simulink model "test_mdl"  (R2018a)
settings: Solver=VariableStepAuto  StartTime=0.0  StopTime=10.0  RelTol=1e-3
(part 7 of 8)

== system test_mdl/FD1_CAN_P702_GASD_MY21_DCV_V06/PCM_HEV/Cluster_HEV_Data5 ==
  HybMdeStat_D_Dsply : Constant
  PlgActvArb_B_Dsply : Constant
  bus_creator : BusCreator  Inputs=2
  port : Outport
  wires:
  bus_creator/1 -> port/1  "Cluster_HEV_Data5"
  HybMdeStat_D_Dsply/1 -> bus_creator/1  "HybMdeStat_D_Dsply"
  PlgActvArb_B_Dsply/1 -> bus_creator/2  "PlgActvArb_B_Dsply"

== system test_mdl/FD1_CAN_P702_GASD_MY21_DCV_V06/PCM_HEV/DCACA_Data4 ==
  DcacElPw_D_Stat : Constant
  DcacEngOnMsgTxt_D_Rq : Constant
  DcacFaltMsgTxt_D_Rq : Constant
  DcacGfciTest_B_Rq : Constant
  DcacHw_D_Confg : Constant
  DcacLedCtl_D_Rq : Constant
  DcacLoFuelMsgTxt_D_Rq : Constant
  DcacOn_B_Rq : Constant
  DcacOut1_Pw_Dsply : Constant
  DcacOut2_Pw_Dsply : Constant
  DcacOut_Pw_DsplyMx : Constant
  DcacSys_B_Falt : Constant
  PwBedPnlEnbl_B_Rq : Constant
  bus_creator : BusCreator  Inputs=13
  port : Outport
  wires:
  bus_creator/1 -> port/1  "DCACA_Data4"
  DcacElPw_D_Stat/1 -> bus_creator/1  "DcacElPw_D_Stat"
  DcacEngOnMsgTxt_D_Rq/1 -> bus_creator/2  "DcacEngOnMsgTxt_D_Rq"
  DcacFaltMsgTxt_D_Rq/1 -> bus_creator/3  "DcacFaltMsgTxt_D_Rq"
  DcacGfciTest_B_Rq/1 -> bus_creator/4  "DcacGfciTest_B_Rq"
  DcacHw_D_Confg/1 -> bus_creator/5  "DcacHw_D_Confg"
  DcacLedCtl_D_Rq/1 -> bus_creator/6  "DcacLedCtl_D_Rq"
  DcacLoFuelMsgTxt_D_Rq/1 -> bus_creator/7  "DcacLoFuelMsgTxt_D_Rq"
  DcacOn_B_Rq/1 -> bus_creator/8  "DcacOn_B_Rq"
  DcacOut1_Pw_Dsply/1 -> bus_creator/9  "DcacOut1_Pw_Dsply"
  DcacOut2_Pw_Dsply/1 -> bus_creator/10  "DcacOut2_Pw_Dsply"
  DcacOut_Pw_DsplyMx/1 -> bus_creator/11  "DcacOut_Pw_DsplyMx"
  DcacSys_B_Falt/1 -> bus_creator/12  "DcacSys_B_Falt"
  PwBedPnlEnbl_B_Rq/1 -> bus_creator/13  "PwBedPnlEnbl_B_Rq"

== system test_mdl/FD1_CAN_P702_GASD_MY21_DCV_V06/PCM_HEV/EngBrakeData ==
  AccEngStat_D_Actl : Constant
  AccStopMde_D_Rq : Constant
  BPedDrvAppl_D_QF : Constant
  BpedDrvAppl_D_Actl : Constant
  CcMde_D_Actl : Constant
  CcOvrrdActv_B_Actl : Constant
  CcStat_D_Actl : Constant
  CmbbDeny_B_ActlPrpl : Constant
  CmbbEngTqMn_B_Actl : Constant
  EngAout_N_MnAllw : Constant
  PrplTqMnSat_B_Actl : Constant
  Veh_V_DsplyCcSet : Constant
  bus_creator : BusCreator  Inputs=12
  port : Outport
  wires:
  bus_creator/1 -> port/1  "EngBrakeData"
  AccEngStat_D_Actl/1 -> bus_creator/1  "AccEngStat_D_Actl"
  AccStopMde_D_Rq/1 -> bus_creator/2  "AccStopMde_D_Rq"
  BPedDrvAppl_D_QF/1 -> bus_creator/3  "BPedDrvAppl_D_QF"
  BpedDrvAppl_D_Actl/1 -> bus_creator/4  "BpedDrvAppl_D_Actl"
  CcMde_D_Actl/1 -> bus_creator/5  "CcMde_D_Actl"
  CcOvrrdActv_B_Actl/1 -> bus_creator/6  "CcOvrrdActv_B_Actl"
  CcStat_D_Actl/1 -> bus_creator/7  "CcStat_D_Actl"
  CmbbDeny_B_ActlPrpl/1 -> bus_creator/8  "CmbbDeny_B_ActlPrpl"
  CmbbEngTqMn_B_Actl/1 -> bus_creator/9  "CmbbEngTqMn_B_Actl"
  EngAout_N_MnAllw/1 -> bus_creator/10  "EngAout_N_MnAllw"
  PrplTqMnSat_B_Actl/1 -> bus_creator/11  "PrplTqMnSat_B_Actl"
  Veh_V_DsplyCcSet/1 -> bus_creator/12  "Veh_V_DsplyCcSet"

== system test_mdl/FD1_CAN_P702_GASD_MY21_DCV_V06/PCM_HEV/EngVehicleSpThrottle ==
  ApedPosPcActl_D_Qf : Constant
  ApedPosPcActl_No_Cnt : Constant
  ApedPosPcActl_No_Cs : Constant
  ApedPos_PcRate_ActlArb : Constant
  ApedPos_Pc_ActlArb : Constant
  EngAout3_N_Actl : Constant
  EngAoutNActl_D_QF : Constant
  EngAout_N_Actl : Constant
  bus_creator : BusCreator  Inputs=8
  port : Outport
  wires:
  bus_creator/1 -> port/1  "EngVehicleSpThrottle"
  ApedPosPcActl_D_Qf/1 -> bus_creator/1  "ApedPosPcActl_D_Qf"
  ApedPosPcActl_No_Cnt/1 -> bus_creator/2  "ApedPosPcActl_No_Cnt"
  ApedPosPcActl_No_Cs/1 -> bus_creator/3  "ApedPosPcActl_No_Cs"
  ApedPos_PcRate_ActlArb/1 -> bus_creator/4  "ApedPos_PcRate_ActlArb"
  ApedPos_Pc_ActlArb/1 -> bus_creator/5  "ApedPos_Pc_ActlArb"
  EngAout3_N_Actl/1 -> bus_creator/6  "EngAout3_N_Actl"
  EngAoutNActl_D_QF/1 -> bus_creator/7  "EngAoutNActl_D_QF"
  EngAout_N_Actl/1 -> bus_creator/8  "EngAout_N_Actl"

== system test_mdl/FD1_CAN_P702_GASD_MY21_DCV_V06/PCM_HEV/EngVehicleSpThrottle2 ==
  GearRvrse_D_Actl : Constant
  StrtrMtrCtlMsgTxt_D2_Rq : Constant
  StrtrMtrCtlMsgTxt_D_Rq : Constant
  StrtrMtrDlyStrt_B_Stat : Constant
  VehVActlEng_D_Qf : Constant
  VehVActlEng_No_Cnt : Constant
  VehVActlEng_No_Cs : Constant
  VehVTrlrAid_B_Avail : Constant
  Veh_V_ActlEng : Constant
  Veh_V_RqCcSet : Constant
  bus_creator : BusCreator  Inputs=10
  port : Outport
  wires:
  bus_creator/1 -> port/1  "EngVehicleSpThrottle2"
  GearRvrse_D_Actl/1 -> bus_creator/1  "GearRvrse_D_Actl"
  StrtrMtrCtlMsgTxt_D2_Rq/1 -> bus_creator/2  "StrtrMtrCtlMsgTxt_D2_Rq"
  StrtrMtrCtlMsgTxt_D_Rq/1 -> bus_creator/3  "StrtrMtrCtlMsgTxt_D_Rq"
  StrtrMtrDlyStrt_B_Stat/1 -> bus_creator/4  "StrtrMtrDlyStrt_B_Stat"
  VehVActlEng_D_Qf/1 -> bus_creator/5  "VehVActlEng_D_Qf"
  VehVActlEng_No_Cnt/1 -> bus_creator/6  "VehVActlEng_No_Cnt"
  VehVActlEng_No_Cs/1 -> bus_creator/7  "VehVActlEng_No_Cs"
  VehVTrlrAid_B_Avail/1 -> bus_creator/8  "VehVTrlrAid_B_Avail"
  Veh_V_ActlEng/1 -> bus_creator/9  "Veh_V_ActlEng"
  Veh_V_RqCcSet/1 -> bus_creator/10  "Veh_V_RqCcSet"

== system test_mdl/FD1_CAN_P702_GASD_MY21_DCV_V06/PCM_HEV/EngineClimateData ==
  AirAmbTe_D_Qf : Constant
  AirAmb_P_Actl : Constant
  AirAmb_Te_Actl : Constant
  AirAmb_Te_ActlFilt : Constant
  AslChime_B_Rq : Constant
  AslIconDsply_D_Rq : Constant
  DynoMde_B_Cmd : Constant
  EcssLamp_D_RqDsply : Constant
  EngAout_Aa_Actl : Constant
  GasPrtc_D_RqDsply : Constant
  HvacHtrCore2_Te_Actl : Constant
  bus_creator : BusCreator  Inputs=11
  port : Outport
  wires:
  bus_creator/1 -> port/1  "EngineClimateData"
  AirAmbTe_D_Qf/1 -> bus_creator/1  "AirAmbTe_D_Qf"
  AirAmb_P_Actl/1 -> bus_creator/2  "AirAmb_P_Actl"
  AirAmb_Te_Actl/1 -> bus_creator/3  "AirAmb_Te_Actl"
  AirAmb_Te_ActlFilt/1 -> bus_creator/4  "AirAmb_Te_ActlFilt"
  AslChime_B_Rq/1 -> bus_creator/5  "AslChime_B_Rq"
  AslIconDsply_D_Rq/1 -> bus_creator/6  "AslIconDsply_D_Rq"
  DynoMde_B_Cmd/1 -> bus_creator/7  "DynoMde_B_Cmd"
  EcssLamp_D_RqDsply/1 -> bus_creator/8  "EcssLamp_D_RqDsply"
  EngAout_Aa_Actl/1 -> bus_creator/9  "EngAout_Aa_Actl"
  GasPrtc_D_RqDsply/1 -> bus_creator/10  "GasPrtc_D_RqDsply"
  HvacHtrCore2_Te_Actl/1 -> bus_creator/11  "HvacHtrCore2_Te_Actl"

== system test_mdl/FD1_CAN_P702_GASD_MY21_DCV_V06/PCM_HEV/EngineData_1 ==
  SeatWorkSrfc_B_Falt : Constant
  TrnIpcDsplyGear_D_Actl : Constant
  TrnIpcDsplyGear_D_Stat : Constant
  TrnIpcDsplyMde_D_Actl : Constant
  TrnIpcDsplyMde_D_Stat : Constant
  TrnIpcDsplyRng2_D_Actl : Constant
  TrnIpcDsplyRng_D_Stat : Constant
  bus_creator : BusCreator  Inputs=7
  port : Outport
  wires:
  bus_creator/1 -> port/1  "EngineData_1"
  SeatWorkSrfc_B_Falt/1 -> bus_creator/1  "SeatWorkSrfc_B_Falt"
  TrnIpcDsplyGear_D_Actl/1 -> bus_creator/2  "TrnIpcDsplyGear_D_Actl"
  TrnIpcDsplyGear_D_Stat/1 -> bus_creator/3  "TrnIpcDsplyGear_D_Stat"
  TrnIpcDsplyMde_D_Actl/1 -> bus_creator/4  "TrnIpcDsplyMde_D_Actl"
  TrnIpcDsplyMde_D_Stat/1 -> bus_creator/5  "TrnIpcDsplyMde_D_Stat"
  TrnIpcDsplyRng2_D_Actl/1 -> bus_creator/6  "TrnIpcDsplyRng2_D_Actl"
  TrnIpcDsplyRng_D_Stat/1 -> bus_creator/7  "TrnIpcDsplyRng_D_Stat"

== system test_mdl/FD1_CAN_P702_GASD_MY21_DCV_V06/PCM_HEV/EngineData_6 ==
  EngClntTe_D_Qf : Constant
  EngClnt_Te_Actl : Constant
  EngGoutLss_Tq_Est : Constant
  EngOil_Te_Actl : Constant
  EngOvrhtMitgActv_D_Ind : Constant
  bus_creator : BusCreator  Inputs=5
  port : Outport
  wires:
  bus_creator/1 -> port/1  "EngineData_6"
  EngClntTe_D_Qf/1 -> bus_creator/1  "EngClntTe_D_Qf"
  EngClnt_Te_Actl/1 -> bus_creator/2  "EngClnt_Te_Actl"
  EngGoutLss_Tq_Est/1 -> bus_creator/3  "EngGoutLss_Tq_Est"
  EngOil_Te_Actl/1 -> bus_creator/4  "EngOil_Te_Actl"
  EngOvrhtMitgActv_D_Ind/1 -> bus_creator/5  "EngOvrhtMitgActv_D_Ind"

== system test_mdl/FD1_CAN_P702_GASD_MY21_DCV_V06/PCM_HEV/EngineData_7 ==
  AirCondClutch_B_Stats : Constant
  AirCondRec_B_Rq : Constant
  EngOilLife_Pc_Actl : Constant
  EngSrvcRqd_B_Rq : Constant
  FuelFillInlet_B_Dsply : Constant
  FuelFilterLamp_B_Dsply : Constant
  FuelFlw_Vl_Dsply : Constant
  HvacAirFullOut_B_Rq : Constant
  OdoCount : Constant
  bus_creator : BusCreator  Inputs=9
  port : Outport
  wires:
  bus_creator/1 -> port/1  "EngineData_7"
  AirCondClutch_B_Stats/1 -> bus_creator/1  "AirCondClutch_B_Stats"
  AirCondRec_B_Rq/1 -> bus_creator/2  "AirCondRec_B_Rq"
  EngOilLife_Pc_Actl/1 -> bus_creator/3  "EngOilLife_Pc_Actl"
  EngSrvcRqd_B_Rq/1 -> bus_creator/4  "EngSrvcRqd_B_Rq"
  FuelFillInlet_B_Dsply/1 -> bus_creator/5  "FuelFillInlet_B_Dsply"
  FuelFilterLamp_B_Dsply/1 -> bus_creator/6  "FuelFilterLamp_B_Dsply"
  FuelFlw_Vl_Dsply/1 -> bus_creator/7  "FuelFlw_Vl_Dsply"
  HvacAirFullOut_B_Rq/1 -> bus_creator/8  "HvacAirFullOut_B_Rq"
  OdoCount/1 -> bus_creator/9  "OdoCount"

== system test_mdl/FD1_CAN_P702_GASD_MY21_DCV_V06/PCM_HEV/Engine_Clutch_Data ==
  CluPdlPosPcMeas_D_Qf : Constant
  CluPdlPos_Pc_Meas : Constant
  CluPdl_PcRate_Actl : Constant
  EngAoutIdl_N_Ntrl : Constant
  EngAout_N_Dsply : Constant
  bus_creator : BusCreator  Inputs=5
  port : Outport
  wires:
  bus_creator/1 -> port/1  "Engine_Clutch_Data"
  CluPdlPosPcMeas_D_Qf/1 -> bus_creator/1  "CluPdlPosPcMeas_D_Qf"
  CluPdlPos_Pc_Meas/1 -> bus_creator/2  "CluPdlPos_Pc_Meas"
  CluPdl_PcRate_Actl/1 -> bus_creator/3  "CluPdl_PcRate_Actl"
  EngAoutIdl_N_Ntrl/1 -> bus_creator/4  "EngAoutIdl_N_Ntrl"
  EngAout_N_Dsply/1 -> bus_creator/5  "EngAout_N_Dsply"

== system test_mdl/FD1_CAN_P702_GASD_MY21_DCV_V06/PCM_HEV/Gear_Shift_by_Wire_3 ==
  GearSelLck_D_Rq : Constant
  PrkBrkActv_D_RqTrnGear : Constant
  TrnCmdCnt_B_Actl : Constant
  TrnCmdState_B_Actl : Constant
  TrnDtpCmd_D_Actl : Constant
  TrnGearCmd_No_Cnt : Constant
  TrnGearCmd_No_Cs : Constant
  TrnGearCmd_Pc_ActlPt : Constant
  TrnGearMsgTxt_D_Rq : Constant
  TrnGearNtmAllow_B_Stat : Constant
  TrnGear_D_RqPt : Constant
  TrnLvrV_D_Rq : Constant
  TrnNtrlTowCmd_D_Actl : Constant
  TrnSbwSysHlth_D_Actl : Constant
  TrnValidGear_D_Cnfm : Constant
  bus_creator : BusCreator  Inputs=15
  port : Outport
  wires:
  bus_creator/1 -> port/1  "Gear_Shift_by_Wire_3"
  GearSelLck_D_Rq/1 -> bus_creator/1  "GearSelLck_D_Rq"
  PrkBrkActv_D_RqTrnGear/1 -> bus_creator/2  "PrkBrkActv_D_RqTrnGear"
  TrnCmdCnt_B_Actl/1 -> bus_creator/3  "TrnCmdCnt_B_Actl"
  TrnCmdState_B_Actl/1 -> bus_creator/4  "TrnCmdState_B_Actl"
  TrnDtpCmd_D_Actl/1 -> bus_creator/5  "TrnDtpCmd_D_Actl"
  TrnGearCmd_No_Cnt/1 -> bus_creator/6  "TrnGearCmd_No_Cnt"
  TrnGearCmd_No_Cs/1 -> bus_creator/7  "TrnGearCmd_No_Cs"
  TrnGearCmd_Pc_ActlPt/1 -> bus_creator/8  "TrnGearCmd_Pc_ActlPt"
  TrnGearMsgTxt_D_Rq/1 -> bus_creator/9  "TrnGearMsgTxt_D_Rq"
  TrnGearNtmAllow_B_Stat/1 -> bus_creator/10  "TrnGearNtmAllow_B_Stat"
  TrnGear_D_RqPt/1 -> bus_creator/11  "TrnGear_D_RqPt"
  TrnLvrV_D_Rq/1 -> bus_creator/12  "TrnLvrV_D_Rq"
  TrnNtrlTowCmd_D_Actl/1 -> bus_creator/13  "TrnNtrlTowCmd_D_Actl"
  TrnSbwSysHlth_D_Actl/1 -> bus_creator/14  "TrnSbwSysHlth_D_Actl"
  TrnValidGear_D_Cnfm/1 -> bus_creator/15  "TrnValidGear_D_Cnfm"

== system test_mdl/FD1_CAN_P702_GASD_MY21_DCV_V06/PCM_HEV/Global_PATS_TargetInfo ==
  bus_creator : BusCreator  Inputs=3
  immoTarget1Cmd : Constant
  immoTarget1Data : Constant
  immoTarget1Status : Constant
  port : Outport
  wires:
  bus_creator/1 -> port/1  "Global_PATS_TargetInfo"
  immoTarget1Cmd/1 -> bus_creator/1  "immoTarget1Cmd"
  immoTarget1Data/1 -> bus_creator/2  "immoTarget1Data"
  immoTarget1Status/1 -> bus_creator/3  "immoTarget1Status"

== system test_mdl/FD1_CAN_P702_GASD_MY21_DCV_V06/PCM_HEV/HEV_Powertrain_Data ==
  HtrnWarnLamp_B_Dsply : Constant
  HybPwLimOn_B_Stat : Constant
  PwPckTqRdy_B_Dsply : Constant
  bus_creator : BusCreator  Inputs=3
  port : Outport
  wires:
  bus_creator/1 -> port/1  "HEV_Powertrain_Data"
  HtrnWarnLamp_B_Dsply/1 -> bus_creator/1  "HtrnWarnLamp_B_Dsply"
  HybPwLimOn_B_Stat/1 -> bus_creator/2  "HybPwLimOn_B_Stat"
  PwPckTqRdy_B_Dsply/1 -> bus_creator/3  "PwPckTqRdy_B_Dsply"

== system test_mdl/FD1_CAN_P702_GASD_MY21_DCV_V06/PCM_HEV/HEV_Powertrain_Data2 ==
  BattTracCnnct_D_Rq : Constant
  PrplTqMnRgen_B_Actl : Constant
  WhlDirAvgDrv_D_Actl : Constant
  bus_creator : BusCreator  Inputs=3
  port : Outport
  wires:
  bus_creator/1 -> port/1  "HEV_Powertrain_Data2"
  BattTracCnnct_D_Rq/1 -> bus_creator/1  "BattTracCnnct_D_Rq"
  PrplTqMnRgen_B_Actl/1 -> bus_creator/2  "PrplTqMnRgen_B_Actl"
  WhlDirAvgDrv_D_Actl/1 -> bus_creator/3  "WhlDirAvgDrv_D_Actl"

== system test_mdl/FD1_CAN_P702_GASD_MY21_DCV_V06/PCM_HEV/HEV_Powertrain_Data6 ==
  BattTracDiagClr_B_Stat : Constant
  DcdcOn_B_Rq : Constant
  EngTeHi_B_Actl : Constant
  ULoBattSpprtSustn_B_Rq : Constant
  VehElEff_No_Avg : Constant
  bus_creator : BusCreator  Inputs=5
  port : Outport
  wires:
  bus_creator/1 -> port/1  "HEV_Powertrain_Data6"
  BattTracDiagClr_B_Stat/1 -> bus_creator/1  "BattTracDiagClr_B_Stat"
  DcdcOn_B_Rq/1 -> bus_creator/2  "DcdcOn_B_Rq"
  EngTeHi_B_Actl/1 -> bus_creator/3  "EngTeHi_B_Actl"
  ULoBattSpprtSustn_B_Rq/1 -> bus_creator/4  "ULoBattSpprtSustn_B_Rq"
  VehElEff_No_Avg/1 -> bus_creator/5  "VehElEff_No_Avg"

== system test_mdl/FD1_CAN_P702_GASD_MY21_DCV_V06/PCM_HEV/HEV_Powertrain_Data7_FD1 ==
  PwFlwBattClimt_B_Dsply : Constant
  PwFlwBatt_D_Dsply : Constant
  PwFlwFuelBatt_B_Dsply : Constant
  PwFlwFuelClimt_B_Dsply : Constant
  PwFlwFuelDrv_D_Dsply : Constant
  RngImpctClim_L_Dsply : Constant
  RngImpctDrv_L_Dsply : Constant
  VehElEffAvg_No_Dsply : Constant
  bus_creator : BusCreator  Inputs=8
  port : Outport
  wires:
  bus_creator/1 -> port/1  "HEV_Powertrain_Data7_FD1"
  PwFlwBattClimt_B_Dsply/1 -> bus_creator/1  "PwFlwBattClimt_B_Dsply"
  PwFlwBatt_D_Dsply/1 -> bus_creator/2  "PwFlwBatt_D_Dsply"
  PwFlwFuelBatt_B_Dsply/1 -> bus_creator/3  "PwFlwFuelBatt_B_Dsply"
  PwFlwFuelClimt_B_Dsply/1 -> bus_creator/4  "PwFlwFuelClimt_B_Dsply"
  PwFlwFuelDrv_D_Dsply/1 -> bus_creator/5  "PwFlwFuelDrv_D_Dsply"
  RngImpctClim_L_Dsply/1 -> bus_creator/6  "RngImpctClim_L_Dsply"
  RngImpctDrv_L_Dsply/1 -> bus_creator/7  "RngImpctDrv_L_Dsply"
  VehElEffAvg_No_Dsply/1 -> bus_creator/8  "VehElEffAvg_No_Dsply"

== system test_mdl/FD1_CAN_P702_GASD_MY21_DCV_V06/PCM_HEV/HEV_Powertrain_Data8_FD1 ==
  ElVehLaterMde_D_Stat : Constant
  ElVehNowMde_D_Stat : Constant
  bus_creator : BusCreator  Inputs=2
  port : Outport
  wires:
  bus_creator/1 -> port/1  "HEV_Powertrain_Data8_FD1"
  ElVehLaterMde_D_Stat/1 -> bus_creator/1  "ElVehLaterMde_D_Stat"
  ElVehNowMde_D_Stat/1 -> bus_creator/2  "ElVehNowMde_D_Stat"

== system test_mdl/FD1_CAN_P702_GASD_MY21_DCV_V06/PCM_HEV/MtrTrac_Data2_FD1 ==
  ChrgStat_D_ActlMntr : Constant
  HybVehMde_D_ActlMntr : Constant
  Inv1Ain_I_ActlMntr : Constant
  Mtr2State_D_ActlMntr : Constant
  VehElRnge_L_Dsply : Constant
  bus_creator : BusCreator  Inputs=5
  port : Outport
  wires:
  bus_creator/1 -> port/1  "MtrTrac_Data2_FD1"
  ChrgStat_D_ActlMntr/1 -> bus_creator/1  "ChrgStat_D_ActlMntr"
  HybVehMde_D_ActlMntr/1 -> bus_creator/2  "HybVehMde_D_ActlMntr"
  Inv1Ain_I_ActlMntr/1 -> bus_creator/3  "Inv1Ain_I_ActlMntr"
  Mtr2State_D_ActlMntr/1 -> bus_creator/4  "Mtr2State_D_ActlMntr"
  VehElRnge_L_Dsply/1 -> bus_creator/5  "VehElRnge_L_Dsply"

== system test_mdl/FD1_CAN_P702_GASD_MY21_DCV_V06/PCM_HEV/OTAPhysPCMtoGWM_ECG ==
  OTAPhysPCMtoGWM_ECG : Constant
  bus_creator : BusCreator  Inputs=1
  port : Outport
  wires:
  bus_creator/1 -> port/1  "OTAPhysPCMtoGWM_ECG"
  OTAPhysPCMtoGWM_ECG/1 -> bus_creator/1  "OTAPhysPCMtoGWM_ECG"

== system test_mdl/FD1_CAN_P702_GASD_MY21_DCV_V06/PCM_HEV/PARSEDPhysPCMtoGWM_ECG ==
  PARSEDPhysPCMtoGWM_ECG : Constant
  bus_creator : BusCreator  Inputs=1
  port : Outport
  wires:
  bus_creator/1 -> port/1  "PARSEDPhysPCMtoGWM_ECG"
  PARSEDPhysPCMtoGWM_ECG/1 -> bus_creator/1  "PARSEDPhysPCMtoGWM_ECG"

== system test_mdl/FD1_CAN_P702_GASD_MY21_DCV_V06/PCM_HEV/PARSEDPushPCMtoGWM_ECG ==
  PARSEDPushPCMtoGWM_ECG : Constant
  bus_creator : BusCreator  Inputs=1
  port : Outport
  wires:
  bus_creator/1 -> port/1  "PARSEDPushPCMtoGWM_ECG"
  PARSEDPushPCMtoGWM_ECG/1 -> bus_creator/1  "PARSEDPushPCMtoGWM_ECG"

== system test_mdl/FD1_CAN_P702_GASD_MY21_DCV_V06/PCM_HEV/PCM_AutoSar_NetworkMgmt ==
  PCM_AutoSarNMControl : Constant
  PCM_AutoSarNMNodeId : Constant
  PCM_AutoSarNMReserved{1..4} (4 alike) : Constant
  PCM_GWNMProxy : Constant
  PCM_GWOnBoardTester : Constant
  bus_creator : BusCreator  Inputs=8
  port : Outport
  wires:
  bus_creator/1 -> port/1  "PCM_AutoSar_NetworkMgmt"
  PCM_AutoSarNMControl/1 -> bus_creator/1  "PCM_AutoSarNMControl"
  PCM_AutoSarNMNodeId/1 -> bus_creator/2  "PCM_AutoSarNMNodeId"
  PCM_AutoSarNMReserved1/1 -> bus_creator/3  "PCM_AutoSarNMReserved1"
  PCM_AutoSarNMReserved2/1 -> bus_creator/4  "PCM_AutoSarNMReserved2"
  PCM_AutoSarNMReserved3/1 -> bus_creator/5  "PCM_AutoSarNMReserved3"
  PCM_AutoSarNMReserved4/1 -> bus_creator/6  "PCM_AutoSarNMReserved4"
  PCM_GWNMProxy/1 -> bus_creator/7  "PCM_GWNMProxy"
  PCM_GWOnBoardTester/1 -> bus_creator/8  "PCM_GWOnBoardTester"

== system test_mdl/FD1_CAN_P702_GASD_MY21_DCV_V06/PCM_HEV/PCM_Rapid_Data_Response_1 ==
  UUDTPCMResponse1 : Constant
  bus_creator : BusCreator  Inputs=1
  port : Outport
  wires:
  bus_creator/1 -> port/1  "PCM_Rapid_Data_Response_1"
  UUDTPCMResponse1/1 -> bus_creator/1  "UUDTPCMResponse1"

== system test_mdl/FD1_CAN_P702_GASD_MY21_DCV_V06/PCM_HEV/PCM_Rapid_Data_Response_2 ==
  UUDTPCMResponse2 : Constant
  bus_creator : BusCreator  Inputs=1
  port : Outport
  wires:
  bus_creator/1 -> port/1  "PCM_Rapid_Data_Response_2"
  UUDTPCMResponse2/1 -> bus_creator/1  "UUDTPCMResponse2"

== system test_mdl/FD1_CAN_P702_GASD_MY21_DCV_V06/PCM_HEV/PowertrainData_1 ==
  AirCondFluidHi_P_Actl : Constant
  CoolantFanStepAct : Constant
  ECMMILRequest : Constant
  EngIdlShutDown_D_Stat : Constant
  EngIdlShutDwnTxt_D_Rq : Constant
  FUEL_ALCOHOL_PERCNT : Constant
  FohEng_D_Rq : Constant
  OilPressureWarning : Constant
  TrnTotLss_Tq_Est : Constant
  TrnTotTq_Rt_Est : Constant
  VehVLimActv_B_Actl : Constant
  VehVLimStat_D_Actl : Constant
  bus_creator : BusCreator  Inputs=12
  port : Outport
  wires:
  bus_creator/1 -> port/1  "PowertrainData_1"
  AirCondFluidHi_P_Actl/1 -> bus_creator/1  "AirCondFluidHi_P_Actl"
  CoolantFanStepAct/1 -> bus_creator/2  "CoolantFanStepAct"
  ECMMILRequest/1 -> bus_creator/3  "ECMMILRequest"
  EngIdlShutDown_D_Stat/1 -> bus_creator/4  "EngIdlShutDown_D_Stat"
  EngIdlShutDwnTxt_D_Rq/1 -> bus_creator/5  "EngIdlShutDwnTxt_D_Rq"
  FUEL_ALCOHOL_PERCNT/1 -> bus_creator/6  "FUEL_ALCOHOL_PERCNT"
  FohEng_D_Rq/1 -> bus_creator/7  "FohEng_D_Rq"
  OilPressureWarning/1 -> bus_creator/8  "OilPressureWarning"
  TrnTotLss_Tq_Est/1 -> bus_creator/9  "TrnTotLss_Tq_Est"
  TrnTotTq_Rt_Est/1 -> bus_creator/10  "TrnTotTq_Rt_Est"
  VehVLimActv_B_Actl/1 -> bus_creator/11  "VehVLimActv_B_Actl"
  VehVLimStat_D_Actl/1 -> bus_creator/12  "VehVLimStat_D_Actl"

== system test_mdl/FD1_CAN_P702_GASD_MY21_DCV_V06/PCM_HEV/PowertrainData_10 ==
  GearEngag_D_Actl : Constant
  GearLvr_D_ActlDrv : Constant
  GearPos_D_Actl : Constant
  GearPos_D_Trg : Constant
  GearPos_No_Cnt : Constant
  GearPos_No_Cs : Constant
  TrnIgnOffDly_T_Rq : Constant
  TrnPrkSys_D_Actl : Constant
  TrnRng_D_Rq : Constant
  bus_creator : BusCreator  Inputs=9
  port : Outport
  wires:
  bus_creator/1 -> port/1  "PowertrainData_10"
  GearEngag_D_Actl/1 -> bus_creator/1  "GearEngag_D_Actl"
  GearLvr_D_ActlDrv/1 -> bus_creator/2  "GearLvr_D_ActlDrv"
  GearPos_D_Actl/1 -> bus_creator/3  "GearPos_D_Actl"
  GearPos_D_Trg/1 -> bus_creator/4  "GearPos_D_Trg"
  GearPos_No_Cnt/1 -> bus_creator/5  "GearPos_No_Cnt"
  GearPos_No_Cs/1 -> bus_creator/6  "GearPos_No_Cs"
  TrnIgnOffDly_T_Rq/1 -> bus_creator/7  "TrnIgnOffDly_T_Rq"
  TrnPrkSys_D_Actl/1 -> bus_creator/8  "TrnPrkSys_D_Actl"
  TrnRng_D_Rq/1 -> bus_creator/9  "TrnRng_D_Rq"

== system test_mdl/FD1_CAN_P702_GASD_MY21_DCV_V06/PCM_HEV/PowertrainData_2 ==
  ApedPos_Pc_ActlDiag : Constant
  EngAirIn_Te_Actl : Constant
  EngClnt_Te_ActlDiag : Constant
  EngLoad_Pc_CalcDiag : Constant
  EngMsgTxt_D_Rq : Constant
  GrllShtrPos_B_Falt : Constant
  GrllShtrPos_D_Cmd : Constant
  IsaOffst_D_Stat : Constant
  ObdWarmUp_B_Complt : Constant
  SlMde_D_RqDsply : Constant
  SlMde_D_Stat : Constant
  bus_creator : BusCreator  Inputs=11
  port : Outport
  wires:
  bus_creator/1 -> port/1  "PowertrainData_2"
  ApedPos_Pc_ActlDiag/1 -> bus_creator/1  "ApedPos_Pc_ActlDiag"
  EngAirIn_Te_Actl/1 -> bus_creator/2  "EngAirIn_Te_Actl"
  EngClnt_Te_ActlDiag/1 -> bus_creator/3  "EngClnt_Te_ActlDiag"
  EngLoad_Pc_CalcDiag/1 -> bus_creator/4  "EngLoad_Pc_CalcDiag"
  EngMsgTxt_D_Rq/1 -> bus_creator/5  "EngMsgTxt_D_Rq"
  GrllShtrPos_B_Falt/1 -> bus_creator/6  "GrllShtrPos_B_Falt"
  GrllShtrPos_D_Cmd/1 -> bus_creator/7  "GrllShtrPos_D_Cmd"
  IsaOffst_D_Stat/1 -> bus_creator/8  "IsaOffst_D_Stat"
  ObdWarmUp_B_Complt/1 -> bus_creator/9  "ObdWarmUp_B_Complt"
  SlMde_D_RqDsply/1 -> bus_creator/10  "SlMde_D_RqDsply"
  SlMde_D_Stat/1 -> bus_creator/11  "SlMde_D_Stat"

== system test_mdl/FD1_CAN_P702_GASD_MY21_DCV_V06/PCM_HEV/PowertrainData_3 ==
  BattULoChrg_U_Cmd : Constant
  ElLoadCtl_D_Rq : Constant
  EngMnfld_P_Actl : Constant
  FuelPumpPwr_B_Rq : Constant
  bus_creator : BusCreator  Inputs=4
  port : Outport
  wires:
  bus_creator/1 -> port/1  "PowertrainData_3"
  BattULoChrg_U_Cmd/1 -> bus_creator/1  "BattULoChrg_U_Cmd"
  ElLoadCtl_D_Rq/1 -> bus_creator/2  "ElLoadCtl_D_Rq"
  EngMnfld_P_Actl/1 -> bus_creator/3  "EngMnfld_P_Actl"
  FuelPumpPwr_B_Rq/1 -> bus_creator/4  "FuelPumpPwr_B_Rq"

== system test_mdl/FD1_CAN_P702_GASD_MY21_DCV_V06/PCM_HEV/PowertrainData_6 ==
  BrkTot_Tq_RqFapLc : Constant
  FapLc_B_Err : Constant
  TrnAin_Pc_RqDrv : Constant
  bus_creator : BusCreator  Inputs=3
  port : Outport
  wires:
  bus_creator/1 -> port/1  "PowertrainData_6"
  BrkTot_Tq_RqFapLc/1 -> bus_creator/1  "BrkTot_Tq_RqFapLc"
  FapLc_B_Err/1 -> bus_creator/2  "FapLc_B_Err"
  TrnAin_Pc_RqDrv/1 -> bus_creator/3  "TrnAin_Pc_RqDrv"

== system test_mdl/FD1_CAN_P702_GASD_MY21_DCV_V06/PCM_HEV/PowertrainData_7 ==
  EcoCochA_Pc_Dsply : Constant
  EcoCochCrus_Pc_Dsply : Constant
  EcoCochDecel_Pc_Dsply : Constant
  EcoCochIdlFuel_Pc_Dsply : Constant
  EcoCochInstNeg_B_Dsply : Constant
  EcoCochInst_Pc_Dsply : Constant
  EcoCochShif_Pc_Dsply : Constant
  bus_creator : BusCreator  Inputs=7
  port : Outport
  wires:
  bus_creator/1 -> port/1  "PowertrainData_7"
  EcoCochA_Pc_Dsply/1 -> bus_creator/1  "EcoCochA_Pc_Dsply"
  EcoCochCrus_Pc_Dsply/1 -> bus_creator/2  "EcoCochCrus_Pc_Dsply"
  EcoCochDecel_Pc_Dsply/1 -> bus_creator/3  "EcoCochDecel_Pc_Dsply"
  EcoCochIdlFuel_Pc_Dsply/1 -> bus_creator/4  "EcoCochIdlFuel_Pc_Dsply"
  EcoCochInstNeg_B_Dsply/1 -> bus_creator/5  "EcoCochInstNeg_B_Dsply"
  EcoCochInst_Pc_Dsply/1 -> bus_creator/6  "EcoCochInst_Pc_Dsply"
  EcoCochShif_Pc_Dsply/1 -> bus_creator/7  "EcoCochShif_Pc_Dsply"

== system test_mdl/FD1_CAN_P702_GASD_MY21_DCV_V06/PCM_HEV/PowertrainData_9 ==
  AutoTowActv_B_Stat : Constant
  AutoTowAllw_D_StatMnu : Constant
  EngExhMdeQuiet_D2_Stat : Constant
  GrossTrainWeight_M_Est : Constant
  HvacCmprLim_D_Stat : Constant
  TrailCtlPt_B_Falt : Constant
  Veh_V_DsplyTrailCtlSet : Constant
  WakeAlarm1_B_Typ : Constant
  WakeAlarm1_T_Rq : Constant
  bus_creator : BusCreator  Inputs=9
  port : Outport
  wires:
  bus_creator/1 -> port/1  "PowertrainData_9"
  AutoTowActv_B_Stat/1 -> bus_creator/1  "AutoTowActv_B_Stat"
  AutoTowAllw_D_StatMnu/1 -> bus_creator/2  "AutoTowAllw_D_StatMnu"
  EngExhMdeQuiet_D2_Stat/1 -> bus_creator/3  "EngExhMdeQuiet_D2_Stat"
  GrossTrainWeight_M_Est/1 -> bus_creator/4  "GrossTrainWeight_M_Est"
  HvacCmprLim_D_Stat/1 -> bus_creator/5  "HvacCmprLim_D_Stat"
  TrailCtlPt_B_Falt/1 -> bus_creator/6  "TrailCtlPt_B_Falt"
  Veh_V_DsplyTrailCtlSet/1 -> bus_creator/7  "Veh_V_DsplyTrailCtlSet"
  WakeAlarm1_B_Typ/1 -> bus_creator/8  "WakeAlarm1_B_Typ"
  WakeAlarm1_T_Rq/1 -> bus_creator/9  "WakeAlarm1_T_Rq"

== system test_mdl/FD1_CAN_P702_GASD_MY21_DCV_V06/PCM_HEV/Powertrain_Data_4 ==
  BpedDrvMsgTxt_B_Dsply : Constant
  FuelLvlWarn_D_ActlEng : Constant
  FuelLvl_Pc_DsplyEng : Constant
  FuelRange_L_DsplyEng : Constant
  RearDiffOilTeWarn_B_Rq : Constant
  RearDiffOil_Te_Actl : Constant
  SelDrvMdePt_D_Stat : Constant
  bus_creator : BusCreator  Inputs=7
  port : Outport
  wires:
  bus_creator/1 -> port/1  "Powertrain_Data_4"
  BpedDrvMsgTxt_B_Dsply/1 -> bus_creator/1  "BpedDrvMsgTxt_B_Dsply"
  FuelLvlWarn_D_ActlEng/1 -> bus_creator/2  "FuelLvlWarn_D_ActlEng"
  FuelLvl_Pc_DsplyEng/1 -> bus_creator/3  "FuelLvl_Pc_DsplyEng"
  FuelRange_L_DsplyEng/1 -> bus_creator/4  "FuelRange_L_DsplyEng"
  RearDiffOilTeWarn_B_Rq/1 -> bus_creator/5  "RearDiffOilTeWarn_B_Rq"
  RearDiffOil_Te_Actl/1 -> bus_creator/6  "RearDiffOil_Te_Actl"
  SelDrvMdePt_D_Stat/1 -> bus_creator/7  "SelDrvMdePt_D_Stat"

== system test_mdl/FD1_CAN_P702_GASD_MY21_DCV_V06/PCM_HEV/Powertrain_Data_5 ==
  AdasLcObtclAbrt_B_Stat : Constant
  AirDamPos_D_Stat : Constant
  BattRgenLoChrg_D_RqEng : Constant
  BattRgenLoDChrg_D_RqEng : Constant
  FapLcActv_B_Stat : Constant
  FapLcInhbt_B_Rq : Constant
  FapLcMaxGrdAbrt_B_Stat : Constant
  FapLcMaxGrdInhbt_B_Stat : Constant
  FapLcObstcl_B_Stat : Constant
  FapLcPrchgBrk_B_Rq : Constant
  FapLcStopHold_B_Rq : Constant
  bus_creator : BusCreator  Inputs=11
  port : Outport
  wires:
  bus_creator/1 -> port/1  "Powertrain_Data_5"
  AdasLcObtclAbrt_B_Stat/1 -> bus_creator/1  "AdasLcObtclAbrt_B_Stat"
  AirDamPos_D_Stat/1 -> bus_creator/2  "AirDamPos_D_Stat"
  BattRgenLoChrg_D_RqEng/1 -> bus_creator/3  "BattRgenLoChrg_D_RqEng"
  BattRgenLoDChrg_D_RqEng/1 -> bus_creator/4  "BattRgenLoDChrg_D_RqEng"
  FapLcActv_B_Stat/1 -> bus_creator/5  "FapLcActv_B_Stat"
  FapLcInhbt_B_Rq/1 -> bus_creator/6  "FapLcInhbt_B_Rq"
  FapLcMaxGrdAbrt_B_Stat/1 -> bus_creator/7  "FapLcMaxGrdAbrt_B_Stat"
  FapLcMaxGrdInhbt_B_Stat/1 -> bus_creator/8  "FapLcMaxGrdInhbt_B_Stat"
  FapLcObstcl_B_Stat/1 -> bus_creator/9  "FapLcObstcl_B_Stat"
  FapLcPrchgBrk_B_Rq/1 -> bus_creator/10  "FapLcPrchgBrk_B_Rq"
  FapLcStopHold_B_Rq/1 -> bus_creator/11  "FapLcStopHold_B_Rq"

== system test_mdl/FD1_CAN_P702_GASD_MY21_DCV_V06/PCM_HEV/Stop_Start ==
  AutoStopPtDelta_I_Est : Constant
  HiElPwInhbt_B_Stat : Constant
  OdoTripVerify_L_Actl : Constant
  StopStrtDrvMde_D_Indic : Constant
  StopStrtIODTxt_D_Rq : Constant
  StopStrtMsgTxt_D_Rq : Constant
  StopStrtStdby_D_Indic : Constant
  bus_creator : BusCreator  Inputs=7
  port : Outport
  wires:
  bus_creator/1 -> port/1  "Stop_Start"
  AutoStopPtDelta_I_Est/1 -> bus_creator/1  "AutoStopPtDelta_I_Est"
  HiElPwInhbt_B_Stat/1 -> bus_creator/2  "HiElPwInhbt_B_Stat"
  OdoTripVerify_L_Actl/1 -> bus_creator/3  "OdoTripVerify_L_Actl"
  StopStrtDrvMde_D_Indic/1 -> bus_creator/4  "StopStrtDrvMde_D_Indic"
  StopStrtIODTxt_D_Rq/1 -> bus_creator/5  "StopStrtIODTxt_D_Rq"
  StopStrtMsgTxt_D_Rq/1 -> bus_creator/6  "StopStrtMsgTxt_D_Rq"
  StopStrtStdby_D_Indic/1 -> bus_creator/7  "StopStrtStdby_D_Indic"

== system test_mdl/FD1_CAN_P702_GASD_MY21_DCV_V06/PCM_HEV/TesterPhysicalResPCM ==
  TesterPhysicalResPCM : Constant
  bus_creator : BusCreator  Inputs=1
  port : Outport
  wires:
  bus_creator/1 -> port/1  "TesterPhysicalResPCM"
  TesterPhysicalResPCM/1 -> bus_creator/1  "TesterPhysicalResPCM"

== system test_mdl/FD1_CAN_P702_GASD_MY21_DCV_V06/PCM_HEV/TorqueDataEngFlags ==
  PrplWhlTotTqRq_No_Cnt : Constant
  PrplWhlTotTqRq_No_Cs : Constant
  PrplWhlTot_Tq_LimMn : Constant
  PrplWhlTot_Tq_Rq : Constant
  PtDrvMde_D_Stat : Constant
  bus_creator : BusCreator  Inputs=5
  port : Outport
  wires:
  bus_creator/1 -> port/1  "TorqueDataEngFlags"
  PrplWhlTotTqRq_No_Cnt/1 -> bus_creator/1  "PrplWhlTotTqRq_No_Cnt"
  PrplWhlTotTqRq_No_Cs/1 -> bus_creator/2  "PrplWhlTotTqRq_No_Cs"
  PrplWhlTot_Tq_LimMn/1 -> bus_creator/3  "PrplWhlTot_Tq_LimMn"
  PrplWhlTot_Tq_Rq/1 -> bus_creator/4  "PrplWhlTot_Tq_Rq"
  PtDrvMde_D_Stat/1 -> bus_creator/5  "PtDrvMde_D_Stat"

== system test_mdl/FD1_CAN_P702_GASD_MY21_DCV_V06/PCM_HEV/TransGearData ==
  GboxOil_Te_Actl : Constant
  GearLvrPos_D_Actl : Constant
  SelDrvMdeSwtch_D_Stat3 : Constant
  TrnShifActv_B_Actl : Constant
  TrnSrvcRqd_B_Rq : Constant
  bus_creator : BusCreator  Inputs=5
  port : Outport
  wires:
  bus_creator/1 -> port/1  "TransGearData"
  GboxOil_Te_Actl/1 -> bus_creator/1  "GboxOil_Te_Actl"
  GearLvrPos_D_Actl/1 -> bus_creator/2  "GearLvrPos_D_Actl"
  SelDrvMdeSwtch_D_Stat3/1 -> bus_creator/3  "SelDrvMdeSwtch_D_Stat3"
  TrnShifActv_B_Actl/1 -> bus_creator/4  "TrnShifActv_B_Actl"
  TrnSrvcRqd_B_Rq/1 -> bus_creator/5  "TrnSrvcRqd_B_Rq"

== system test_mdl/FD1_CAN_P702_GASD_MY21_DCV_V06/PCM_HEV/VehicleOperatingModes ==
  ElPw_D_Stat : Constant
  ElPw_D_StatStrtStop : Constant
  Eng_D_Stat : Constant
  PlgActvArb_B_Actl : Constant
  PrplWhlRgenMn_Tq_Actl : Constant
  PrplWhlTot2_Tq_Actl : Constant
  PwPckTq_D_Stat : Constant
  TrnAinTq_D_Qf : Constant
  TrnAin_Tq_Actl : Constant
  bus_creator : BusCreator  Inputs=9
  port : Outport
  wires:
  bus_creator/1 -> port/1  "VehicleOperatingModes"
  ElPw_D_Stat/1 -> bus_creator/1  "ElPw_D_Stat"
  ElPw_D_StatStrtStop/1 -> bus_creator/2  "ElPw_D_StatStrtStop"
  Eng_D_Stat/1 -> bus_creator/3  "Eng_D_Stat"
  PlgActvArb_B_Actl/1 -> bus_creator/4  "PlgActvArb_B_Actl"
  PrplWhlRgenMn_Tq_Actl/1 -> bus_creator/5  "PrplWhlRgenMn_Tq_Actl"
  PrplWhlTot2_Tq_Actl/1 -> bus_creator/6  "PrplWhlTot2_Tq_Actl"
  PwPckTq_D_Stat/1 -> bus_creator/7  "PwPckTq_D_Stat"
  TrnAinTq_D_Qf/1 -> bus_creator/8  "TrnAinTq_D_Qf"
  TrnAin_Tq_Actl/1 -> bus_creator/9  "TrnAin_Tq_Actl"

== system test_mdl/FD1_CAN_P702_GASD_MY21_DCV_V06/PSCM/EPAS_INFO ==
  DrvSteActv_B_Stat : Constant
  DrvSte_Tq_Actl : Constant
  EPAS_Failure : Constant
  SAPPAngleControlStat{1..6} (6 alike) : Constant
  SteMdule_D_Stat : Constant
  SteMdule_I_Est : Constant
  SteMdule_U_Meas : Constant
  SteeringColumnTorque : Constant
  TrlrHitchLamp_D_Rqst : Constant
  VehVTrlrAid_B_Rq : Constant
  Veh_V_RqMxTrlrAid : Constant
  bus_creator : BusCreator  Inputs=16
  port : Outport
  wires:
  bus_creator/1 -> port/1  "EPAS_INFO"
  DrvSteActv_B_Stat/1 -> bus_creator/1  "DrvSteActv_B_Stat"
  DrvSte_Tq_Actl/1 -> bus_creator/2  "DrvSte_Tq_Actl"
  EPAS_Failure/1 -> bus_creator/3  "EPAS_Failure"
  SAPPAngleControlStat1/1 -> bus_creator/4  "SAPPAngleControlStat1"
  SAPPAngleControlStat2/1 -> bus_creator/5  "SAPPAngleControlStat2"
  SAPPAngleControlStat3/1 -> bus_creator/6  "SAPPAngleControlStat3"
  SAPPAngleControlStat4/1 -> bus_creator/7  "SAPPAngleControlStat4"
  SAPPAngleControlStat5/1 -> bus_creator/8  "SAPPAngleControlStat5"
  SAPPAngleControlStat6/1 -> bus_creator/9  "SAPPAngleControlStat6"
  SteMdule_D_Stat/1 -> bus_creator/10  "SteMdule_D_Stat"
  SteMdule_I_Est/1 -> bus_creator/11  "SteMdule_I_Est"
  SteMdule_U_Meas/1 -> bus_creator/12  "SteMdule_U_Meas"
  SteeringColumnTorque/1 -> bus_creator/13  "SteeringColumnTorque"
  TrlrHitchLamp_D_Rqst/1 -> bus_creator/14  "TrlrHitchLamp_D_Rqst"
  VehVTrlrAid_B_Rq/1 -> bus_creator/15  "VehVTrlrAid_B_Rq"
  Veh_V_RqMxTrlrAid/1 -> bus_creator/16  "Veh_V_RqMxTrlrAid"

== system test_mdl/FD1_CAN_P702_GASD_MY21_DCV_V06/PSCM/Lane_Assist_Data3_FD1 ==
  LaActAvail_D_Actl : Constant
  LaActDeny_B_Actl : Constant
  LaHandsOff_B_Actl : Constant
  LatCtlCpbltyDStat_No_Cnt : Constant
  LatCtlCpbltyDStat_No_Cs : Constant
  LatCtlCpblty_D_Stat : Constant
  LatCtlLim_D_Stat : Constant
  LatCtlSte_D_Stat : Constant
  LsmcBrkDecelEnbl_D_Rq : Constant
  LsmcBrk_Tq_Rq : Constant
  TjaHandsOnCnfdnc_B_Est : Constant
  TrlrAn_An_TrgtCalc : Constant
  bus_creator : BusCreator  Inputs=12
  port : Outport
  wires:
  bus_creator/1 -> port/1  "Lane_Assist_Data3_FD1"
  LaActAvail_D_Actl/1 -> bus_creator/1  "LaActAvail_D_Actl"
  LaActDeny_B_Actl/1 -> bus_creator/2  "LaActDeny_B_Actl"
  LaHandsOff_B_Actl/1 -> bus_creator/3  "LaHandsOff_B_Actl"
  LatCtlCpbltyDStat_No_Cnt/1 -> bus_creator/4  "LatCtlCpbltyDStat_No_Cnt"
  LatCtlCpbltyDStat_No_Cs/1 -> bus_creator/5  "LatCtlCpbltyDStat_No_Cs"
  LatCtlCpblty_D_Stat/1 -> bus_creator/6  "LatCtlCpblty_D_Stat"
  LatCtlLim_D_Stat/1 -> bus_creator/7  "LatCtlLim_D_Stat"
  LatCtlSte_D_Stat/1 -> bus_creator/8  "LatCtlSte_D_Stat"
  LsmcBrkDecelEnbl_D_Rq/1 -> bus_creator/9  "LsmcBrkDecelEnbl_D_Rq"
  LsmcBrk_Tq_Rq/1 -> bus_creator/10  "LsmcBrk_Tq_Rq"
  TjaHandsOnCnfdnc_B_Est/1 -> bus_creator/11  "TjaHandsOnCnfdnc_B_Est"
  TrlrAn_An_TrgtCalc/1 -> bus_creator/12  "TrlrAn_An_TrgtCalc"

== system test_mdl/FD1_CAN_P702_GASD_MY21_DCV_V06/PSCM/PSCM_AutoSar_NetwrkMgmt ==
  PSCM_AutoSarNMControl : Constant
  PSCM_AutoSarNMNodeId : Constant
  PSCM_AutoSarNMReserved{1..4} (4 alike) : Constant
  PSCM_GWNMProxy : Constant
  PSCM_GWOnBoardTester : Constant
  bus_creator : BusCreator  Inputs=8
  port : Outport
  wires:
  bus_creator/1 -> port/1  "PSCM_AutoSar_NetwrkMgmt"
  PSCM_AutoSarNMControl/1 -> bus_creator/1  "PSCM_AutoSarNMControl"
  PSCM_AutoSarNMNodeId/1 -> bus_creator/2  "PSCM_AutoSarNMNodeId"
  PSCM_AutoSarNMReserved1/1 -> bus_creator/3  "PSCM_AutoSarNMReserved1"
  PSCM_AutoSarNMReserved2/1 -> bus_creator/4  "PSCM_AutoSarNMReserved2"
  PSCM_AutoSarNMReserved3/1 -> bus_creator/5  "PSCM_AutoSarNMReserved3"
  PSCM_AutoSarNMReserved4/1 -> bus_creator/6  "PSCM_AutoSarNMReserved4"
  PSCM_GWNMProxy/1 -> bus_creator/7  "PSCM_GWNMProxy"
  PSCM_GWOnBoardTester/1 -> bus_creator/8  "PSCM_GWOnBoardTester"

== system test_mdl/FD1_CAN_P702_GASD_MY21_DCV_V06/PSCM/SteeringPinion_Data ==
  StePinAn_No_Cnt : Constant
  StePinAn_No_Cs : Constant
  StePinCompAnEst_D_Qf : Constant
  StePinComp_An_Est : Constant
  StePinRelInit_An_Sns : Constant
  StePw_B_Rq : Constant
  bus_creator : BusCreator  Inputs=6
  port : Outport
  wires:
  bus_creator/1 -> port/1  "SteeringPinion_Data"
  StePinAn_No_Cnt/1 -> bus_creator/1  "StePinAn_No_Cnt"
  StePinAn_No_Cs/1 -> bus_creator/2  "StePinAn_No_Cs"
  StePinCompAnEst_D_Qf/1 -> bus_creator/3  "StePinCompAnEst_D_Qf"
  StePinComp_An_Est/1 -> bus_creator/4  "StePinComp_An_Est"
  StePinRelInit_An_Sns/1 -> bus_creator/5  "StePinRelInit_An_Sns"
  StePw_B_Rq/1 -> bus_creator/6  "StePw_B_Rq"

== system test_mdl/FD1_CAN_P702_GASD_MY21_DCV_V06/PSCM/TesterPhysicalResPSCM ==
  TesterPhysicalResPSCM : Constant
  bus_creator : BusCreator  Inputs=1
  port : Outport
  wires:
  bus_creator/1 -> port/1  "TesterPhysicalResPSCM"
  TesterPhysicalResPSCM/1 -> bus_creator/1  "TesterPhysicalResPSCM"

== system test_mdl/FD1_CAN_P702_GASD_MY21_DCV_V06/PSCM/TrailerAid_Data2 ==
  EsaOn_B_Stat : Constant
  HitchToTrlrAxle_L_Calc : Constant
  SelDrvMdeSte_D_Stat : Constant
  TrlrAidEnbl_D2_Stat : Constant
  TrlrAidMsgTxt_D2_Rq : Constant
  TrlrAidSetup_D2_Stat : Constant
  TrlrAidTrgtId_No_Rq : Constant
  TrlrAidTrlrId_No_Rq : Constant
  TrlrAnOffst_An2_Calc : Constant
  TrlrAn_An_MxCalc : Constant
  TrlrAn_An_WarnCalc : Constant
  bus_creator : BusCreator  Inputs=11
  port : Outport
  wires:
  bus_creator/1 -> port/1  "TrailerAid_Data2"
  EsaOn_B_Stat/1 -> bus_creator/1  "EsaOn_B_Stat"
  HitchToTrlrAxle_L_Calc/1 -> bus_creator/2  "HitchToTrlrAxle_L_Calc"
  SelDrvMdeSte_D_Stat/1 -> bus_creator/3  "SelDrvMdeSte_D_Stat"
  TrlrAidEnbl_D2_Stat/1 -> bus_creator/4  "TrlrAidEnbl_D2_Stat"
  TrlrAidMsgTxt_D2_Rq/1 -> bus_creator/5  "TrlrAidMsgTxt_D2_Rq"
  TrlrAidSetup_D2_Stat/1 -> bus_creator/6  "TrlrAidSetup_D2_Stat"
  TrlrAidTrgtId_No_Rq/1 -> bus_creator/7  "TrlrAidTrgtId_No_Rq"
  TrlrAidTrlrId_No_Rq/1 -> bus_creator/8  "TrlrAidTrlrId_No_Rq"
  TrlrAnOffst_An2_Calc/1 -> bus_creator/9  "TrlrAnOffst_An2_Calc"
  TrlrAn_An_MxCalc/1 -> bus_creator/10  "TrlrAn_An_MxCalc"
  TrlrAn_An_WarnCalc/1 -> bus_creator/11  "TrlrAn_An_WarnCalc"

== system test_mdl/FD1_CAN_P702_GASD_MY21_DCV_V06/SOBDMC_HPCM_FD1/AC_Compressor_Req_FD1 ==
  ElCmprEnbl_B_Rq : Constant
  ElCmpr_N_Rq : Constant
  bus_creator : BusCreator  Inputs=2
  port : Outport
  wires:
  bus_creator/1 -> port/1  "AC_Compressor_Req_FD1"
  ElCmprEnbl_B_Rq/1 -> bus_creator/1  "ElCmprEnbl_B_Rq"
  ElCmpr_N_Rq/1 -> bus_creator/2  "ElCmpr_N_Rq"

== system test_mdl/FD1_CAN_P702_GASD_MY21_DCV_V06/SOBDMC_HPCM_FD1/ChargeSettings_FD1 ==
  ChrgLocIdCurnt_D_Sav : Constant
  ChrgLocIdUnsAck_B_Stat : Constant
  ChrgNowEnbl_B_Saved : Constant
  ChrgPrflWkdy_No_Actl : Constant
  ChrgPrflWknd_No_Actl : Constant
  ChrgProgIdSaved_D_Stat : Constant
  ChrgToPcWkdySav_D_Stat : Constant
  ChrgToPcWkndSav_D_Stat : Constant
  bus_creator : BusCreator  Inputs=8
  port : Outport
  wires:
  bus_creator/1 -> port/1  "ChargeSettings_FD1"
  ChrgLocIdCurnt_D_Sav/1 -> bus_creator/1  "ChrgLocIdCurnt_D_Sav"
  ChrgLocIdUnsAck_B_Stat/1 -> bus_creator/2  "ChrgLocIdUnsAck_B_Stat"
  ChrgNowEnbl_B_Saved/1 -> bus_creator/3  "ChrgNowEnbl_B_Saved"
  ChrgPrflWkdy_No_Actl/1 -> bus_creator/4  "ChrgPrflWkdy_No_Actl"
  ChrgPrflWknd_No_Actl/1 -> bus_creator/5  "ChrgPrflWknd_No_Actl"
  ChrgProgIdSaved_D_Stat/1 -> bus_creator/6  "ChrgProgIdSaved_D_Stat"
  ChrgToPcWkdySav_D_Stat/1 -> bus_creator/7  "ChrgToPcWkdySav_D_Stat"
  ChrgToPcWkndSav_D_Stat/1 -> bus_creator/8  "ChrgToPcWkndSav_D_Stat"

== system test_mdl/FD1_CAN_P702_GASD_MY21_DCV_V06/SOBDMC_HPCM_FD1/Cluster_HEV_Data1_FD1 ==
  ChrgStat_D_Dsply : Constant
  RgenTrip_L_Dsply : Constant
  RgenTrip_Pc_Dsply : Constant
  bus_creator : BusCreator  Inputs=3
  port : Outport
  wires:
  bus_creator/1 -> port/1  "Cluster_HEV_Data1_FD1"
  ChrgStat_D_Dsply/1 -> bus_creator/1  "ChrgStat_D_Dsply"
  RgenTrip_L_Dsply/1 -> bus_creator/2  "RgenTrip_L_Dsply"
  RgenTrip_Pc_Dsply/1 -> bus_creator/3  "RgenTrip_Pc_Dsply"

== system test_mdl/FD1_CAN_P702_GASD_MY21_DCV_V06/SOBDMC_HPCM_FD1/Cluster_HEV_Data4_FD1 ==
  BattChrgCmpltPt_T_Est : Constant
  BattChrgTrgSocPt_T_Est : Constant
  BattChrgTrgtLPt_T_Est : Constant
  BattElecPerf_D_Actl : Constant
  bus_creator : BusCreator  Inputs=4
  port : Outport
  wires:
  bus_creator/1 -> port/1  "Cluster_HEV_Data4_FD1"
  BattChrgCmpltPt_T_Est/1 -> bus_creator/1  "BattChrgCmpltPt_T_Est"
  BattChrgTrgSocPt_T_Est/1 -> bus_creator/2  "BattChrgTrgSocPt_T_Est"
  BattChrgTrgtLPt_T_Est/1 -> bus_creator/3  "BattChrgTrgtLPt_T_Est"
  BattElecPerf_D_Actl/1 -> bus_creator/4  "BattElecPerf_D_Actl"

== system test_mdl/FD1_CAN_P702_GASD_MY21_DCV_V06/SOBDMC_HPCM_FD1/Cluster_HEV_Data5 ==
  HybMdeStat_D_Dsply : Constant
  PlgActvArb_B_Dsply : Constant
  bus_creator : BusCreator  Inputs=2
  port : Outport
  wires:
  bus_creator/1 -> port/1  "Cluster_HEV_Data5"
  HybMdeStat_D_Dsply/1 -> bus_creator/1  "HybMdeStat_D_Dsply"
  PlgActvArb_B_Dsply/1 -> bus_creator/2  "PlgActvArb_B_Dsply"

== system test_mdl/FD1_CAN_P702_GASD_MY21_DCV_V06/SOBDMC_HPCM_FD1/Cluster_HEV_Data7_FD1 ==
  BrkEvntComplt_B_Dsply : Constant
  PreCondStat_D_Dsply : Constant
  RgenEvntLvl_Pc_Dsply : Constant
  bus_creator : BusCreator  Inputs=3
  port : Outport
  wires:
  bus_creator/1 -> port/1  "Cluster_HEV_Data7_FD1"
  BrkEvntComplt_B_Dsply/1 -> bus_creator/1  "BrkEvntComplt_B_Dsply"
  PreCondStat_D_Dsply/1 -> bus_creator/2  "PreCondStat_D_Dsply"
  RgenEvntLvl_Pc_Dsply/1 -> bus_creator/3  "RgenEvntLvl_Pc_Dsply"

== system test_mdl/FD1_CAN_P702_GASD_MY21_DCV_V06/SOBDMC_HPCM_FD1/Cluster_HEV_Data9_FD1 ==
  MtrTrac2_Tq_Actl : Constant
  NtfctnConflict1_D_Rq : Constant
  OfbChrgSetSync_D_Stat : Constant
  PtRmtRprt_D_Rq : Constant
  bus_creator : BusCreator  Inputs=4
  port : Outport
  wires:
  bus_creator/1 -> port/1  "Cluster_HEV_Data9_FD1"
  MtrTrac2_Tq_Actl/1 -> bus_creator/1  "MtrTrac2_Tq_Actl"
  NtfctnConflict1_D_Rq/1 -> bus_creator/2  "NtfctnConflict1_D_Rq"
  OfbChrgSetSync_D_Stat/1 -> bus_creator/3  "OfbChrgSetSync_D_Stat"
  PtRmtRprt_D_Rq/1 -> bus_creator/4  "PtRmtRprt_D_Rq"

== system test_mdl/FD1_CAN_P702_GASD_MY21_DCV_V06/SOBDMC_HPCM_FD1/ConsTip_Data_FD1 ==
  ConsTipV_No_Dsply : Constant
  bus_creator : BusCreator  Inputs=1
  port : Outport
  wires:
  bus_creator/1 -> port/1  "ConsTip_Data_FD1"
  ConsTipV_No_Dsply/1 -> bus_creator/1  "ConsTipV_No_Dsply"

== system test_mdl/FD1_CAN_P702_GASD_MY21_DCV_V06/SOBDMC_HPCM_FD1/GWM_HPCM_i_FrP10_FD1 ==
  ActChrgEndDay_No_Actl : Constant
  ActChrgEndHr_No_Actl : Constant
  ActChrgEndMin_No_Actl : Constant
  ActChrgEndMnth_No_Actl : Constant
  ActChrgEndYr_No2_Actl : Constant
  ActChrgEndYr_No_Actl : Constant
  BattChrgTrgtLMin_T_Est : Constant
  bus_creator : BusCreator  Inputs=7
  port : Outport
  wires:
  bus_creator/1 -> port/1  "GWM_HPCM_i_FrP10_FD1"
  ActChrgEndDay_No_Actl/1 -> bus_creator/1  "ActChrgEndDay_No_Actl"
  ActChrgEndHr_No_Actl/1 -> bus_creator/2  "ActChrgEndHr_No_Actl"
  ActChrgEndMin_No_Actl/1 -> bus_creator/3  "ActChrgEndMin_No_Actl"
  ActChrgEndMnth_No_Actl/1 -> bus_creator/4  "ActChrgEndMnth_No_Actl"
  ActChrgEndYr_No2_Actl/1 -> bus_creator/5  "ActChrgEndYr_No2_Actl"
  ActChrgEndYr_No_Actl/1 -> bus_creator/6  "ActChrgEndYr_No_Actl"
  BattChrgTrgtLMin_T_Est/1 -> bus_creator/7  "BattChrgTrgtLMin_T_Est"

== system test_mdl/FD1_CAN_P702_GASD_MY21_DCV_V06/SOBDMC_HPCM_FD1/GWM_HPCM_i_FrP11_FD1 ==
  ActChrgStrMnth_No_Actl : Constant
  ActChrgStrtDay_No_Actl : Constant
  ActChrgStrtHr_No_Actl : Constant
  ActChrgStrtMin_No_Actl : Constant
  ActChrgStrtYr_No2_Actl : Constant
  ActChrgStrtYr_No_Actl : Constant
  BattChrgTrgtLMax_T_Est : Constant
  bus_creator : BusCreator  Inputs=7
  port : Outport
  wires:
  bus_creator/1 -> port/1  "GWM_HPCM_i_FrP11_FD1"
  ActChrgStrMnth_No_Actl/1 -> bus_creator/1  "ActChrgStrMnth_No_Actl"
  ActChrgStrtDay_No_Actl/1 -> bus_creator/2  "ActChrgStrtDay_No_Actl"
  ActChrgStrtHr_No_Actl/1 -> bus_creator/3  "ActChrgStrtHr_No_Actl"
  ActChrgStrtMin_No_Actl/1 -> bus_creator/4  "ActChrgStrtMin_No_Actl"
  ActChrgStrtYr_No2_Actl/1 -> bus_creator/5  "ActChrgStrtYr_No2_Actl"
  ActChrgStrtYr_No_Actl/1 -> bus_creator/6  "ActChrgStrtYr_No_Actl"
  BattChrgTrgtLMax_T_Est/1 -> bus_creator/7  "BattChrgTrgtLMax_T_Est"

== system test_mdl/FD1_CAN_P702_GASD_MY21_DCV_V06/SOBDMC_HPCM_FD1/Global_PATS_Target2_FD1 ==
  bus_creator : BusCreator  Inputs=3
  immoTarget2Cmd : Constant
  immoTarget2Data : Constant
  immoTarget2Status : Constant
  port : Outport
  wires:
  bus_creator/1 -> port/1  "Global_PATS_Target2_FD1"
  immoTarget2Cmd/1 -> bus_creator/1  "immoTarget2Cmd"
  immoTarget2Data/1 -> bus_creator/2  "immoTarget2Data"
  immoTarget2Status/1 -> bus_creator/3  "immoTarget2Status"

== system test_mdl/FD1_CAN_P702_GASD_MY21_DCV_V06/SOBDMC_HPCM_FD1/GoTimeSettings_FD1 ==
  ChrgGoTAllOn_B_Stat : Constant
  ChrgGoTElement_B_Dsply : Constant
  ChrgGoTElement_D_Stat : Constant
  ChrgGoTExtHtrEnbl_B_Rq : Constant
  ChrgGoTExtHtr_B_Stat : Constant
  ChrgGoTHr_T_Stat : Constant
  ChrgGoTMnte_D_Stat : Constant
  ChrgGoTNext_D_Stat : Constant
  ChrgGoTPrcond_D_Stat : Constant
  ChrgGoTTouchEnbl_B_Rq : Constant
  ChrgGoTTouch_B_Stat : Constant
  ChrgLocIdCurnt_D_Uns : Constant
  bus_creator : BusCreator  Inputs=12
  port : Outport
  wires:
  bus_creator/1 -> port/1  "GoTimeSettings_FD1"
  ChrgGoTAllOn_B_Stat/1 -> bus_creator/1  "ChrgGoTAllOn_B_Stat"
  ChrgGoTElement_B_Dsply/1 -> bus_creator/2  "ChrgGoTElement_B_Dsply"
  ChrgGoTElement_D_Stat/1 -> bus_creator/3  "ChrgGoTElement_D_Stat"
  ChrgGoTExtHtrEnbl_B_Rq/1 -> bus_creator/4  "ChrgGoTExtHtrEnbl_B_Rq"
  ChrgGoTExtHtr_B_Stat/1 -> bus_creator/5  "ChrgGoTExtHtr_B_Stat"
  ChrgGoTHr_T_Stat/1 -> bus_creator/6  "ChrgGoTHr_T_Stat"
  ChrgGoTMnte_D_Stat/1 -> bus_creator/7  "ChrgGoTMnte_D_Stat"
  ChrgGoTNext_D_Stat/1 -> bus_creator/8  "ChrgGoTNext_D_Stat"
  ChrgGoTPrcond_D_Stat/1 -> bus_creator/9  "ChrgGoTPrcond_D_Stat"
  ChrgGoTTouchEnbl_B_Rq/1 -> bus_creator/10  "ChrgGoTTouchEnbl_B_Rq"
  ChrgGoTTouch_B_Stat/1 -> bus_creator/11  "ChrgGoTTouch_B_Stat"
  ChrgLocIdCurnt_D_Uns/1 -> bus_creator/12  "ChrgLocIdCurnt_D_Uns"

== system test_mdl/FD1_CAN_P702_GASD_MY21_DCV_V06/SOBDMC_HPCM_FD1/HEV_ChargeStat_FD1 ==
  ChargeNowDuration_St : Constant
  EstmChrgTimeHP_St : Constant
  EstmChrgTimeLP_St : Constant
  NxtUsgSocEst_Pc_Dsply : Constant
  VehElRngeNut_L_Dsply : Constant
  bus_creator : BusCreator  Inputs=5
  port : Outport
  wires:
  bus_creator/1 -> port/1  "HEV_ChargeStat_FD1"
  ChargeNowDuration_St/1 -> bus_creator/1  "ChargeNowDuration_St"
  EstmChrgTimeHP_St/1 -> bus_creator/2  "EstmChrgTimeHP_St"
  EstmChrgTimeLP_St/1 -> bus_creator/3  "EstmChrgTimeLP_St"
  NxtUsgSocEst_Pc_Dsply/1 -> bus_creator/4  "NxtUsgSocEst_Pc_Dsply"
  VehElRngeNut_L_Dsply/1 -> bus_creator/5  "VehElRngeNut_L_Dsply"

== system test_mdl/FD1_CAN_P702_GASD_MY21_DCV_V06/SOBDMC_HPCM_FD1/MHT_EV_Wakeup_FD1 ==
  BattChlrSov_B_Rq : Constant
  BattChrgTrgtSoC_D_Rq : Constant
  BattTracClntVlv_B_Rq : Constant
  BattTracDrvSustn_B_Rq : Constant
  BrkAppl_D_RqPt : Constant
  CabinDrvSustn_B_Rq : Constant
  CabnEvapSovFront_B_Rq : Constant
  CabnEvapSovRear_B_Rq : Constant
  ChrgNowEvnt_B_Stat : Constant
  HeatCoreSovRear_B_Rq : Constant
  HtrnClntFlw_D_Rq : Constant
  HtrnCnnctPwr_B_Stat : Constant
  HtrnDcdcDis_B_Rq : Constant
  PreCondBatt_B_Actl : Constant
  PtcHtr_D_Stat : Constant
  WakeAlarm0_B_Typ : Constant
  WakeAlarm0_T_Rq : Constant
  bus_creator : BusCreator  Inputs=17
  port : Outport
  wires:
  bus_creator/1 -> port/1  "MHT_EV_Wakeup_FD1"
  BattChlrSov_B_Rq/1 -> bus_creator/1  "BattChlrSov_B_Rq"
  BattChrgTrgtSoC_D_Rq/1 -> bus_creator/2  "BattChrgTrgtSoC_D_Rq"
  BattTracClntVlv_B_Rq/1 -> bus_creator/3  "BattTracClntVlv_B_Rq"
  BattTracDrvSustn_B_Rq/1 -> bus_creator/4  "BattTracDrvSustn_B_Rq"
  BrkAppl_D_RqPt/1 -> bus_creator/5  "BrkAppl_D_RqPt"
  CabinDrvSustn_B_Rq/1 -> bus_creator/6  "CabinDrvSustn_B_Rq"
  CabnEvapSovFront_B_Rq/1 -> bus_creator/7  "CabnEvapSovFront_B_Rq"
  CabnEvapSovRear_B_Rq/1 -> bus_creator/8  "CabnEvapSovRear_B_Rq"
  ChrgNowEvnt_B_Stat/1 -> bus_creator/9  "ChrgNowEvnt_B_Stat"
  HeatCoreSovRear_B_Rq/1 -> bus_creator/10  "HeatCoreSovRear_B_Rq"
  HtrnClntFlw_D_Rq/1 -> bus_creator/11  "HtrnClntFlw_D_Rq"
  HtrnCnnctPwr_B_Stat/1 -> bus_creator/12  "HtrnCnnctPwr_B_Stat"
  HtrnDcdcDis_B_Rq/1 -> bus_creator/13  "HtrnDcdcDis_B_Rq"
  PreCondBatt_B_Actl/1 -> bus_creator/14  "PreCondBatt_B_Actl"
  PtcHtr_D_Stat/1 -> bus_creator/15  "PtcHtr_D_Stat"
  WakeAlarm0_B_Typ/1 -> bus_creator/16  "WakeAlarm0_B_Typ"
  WakeAlarm0_T_Rq/1 -> bus_creator/17  "WakeAlarm0_T_Rq"

== system test_mdl/FD1_CAN_P702_GASD_MY21_DCV_V06/SOBDMC_HPCM_FD1/MtrTracData_1_FD1 ==
  Inv1_Te_Actl : Constant
  Mtr2Aout_W_ActlMntr : Constant
  Mtr2CntlTeAlrm_B_Stat : Constant
  MtrTrac2Coil_Te_Actl : Constant
  MtrTrac2Falt_B_Stat : Constant
  MtrTrac2Inv_Te_Actl : Constant
  MtrTrac2TeAlrm_B_Stat : Constant
  MtrTrac2_I_Actl : Constant
  MtrTrac2_U_Actl : Constant
  bus_creator : BusCreator  Inputs=9
  port : Outport
  wires:
  bus_creator/1 -> port/1  "MtrTracData_1_FD1"
  Inv1_Te_Actl/1 -> bus_creator/1  "Inv1_Te_Actl"
  Mtr2Aout_W_ActlMntr/1 -> bus_creator/2  "Mtr2Aout_W_ActlMntr"
  Mtr2CntlTeAlrm_B_Stat/1 -> bus_creator/3  "Mtr2CntlTeAlrm_B_Stat"
  MtrTrac2Coil_Te_Actl/1 -> bus_creator/4  "MtrTrac2Coil_Te_Actl"
  MtrTrac2Falt_B_Stat/1 -> bus_creator/5  "MtrTrac2Falt_B_Stat"
  MtrTrac2Inv_Te_Actl/1 -> bus_creator/6  "MtrTrac2Inv_Te_Actl"
  MtrTrac2TeAlrm_B_Stat/1 -> bus_creator/7  "MtrTrac2TeAlrm_B_Stat"
  MtrTrac2_I_Actl/1 -> bus_creator/8  "MtrTrac2_I_Actl"
  MtrTrac2_U_Actl/1 -> bus_creator/9  "MtrTrac2_U_Actl"

== system test_mdl/FD1_CAN_P702_GASD_MY21_DCV_V06/SOBDMC_HPCM_FD1/MtrTrac_Data2_FD1 ==
  ChrgStat_D_ActlMntr : Constant
  HybVehMde_D_ActlMntr : Constant
  Inv1Ain_I_ActlMntr : Constant
  Mtr2State_D_ActlMntr : Constant
  VehElRnge_L_Dsply : Constant
  bus_creator : BusCreator  Inputs=5
  port : Outport
  wires:
  bus_creator/1 -> port/1  "MtrTrac_Data2_FD1"
  ChrgStat_D_ActlMntr/1 -> bus_creator/1  "ChrgStat_D_ActlMntr"
  HybVehMde_D_ActlMntr/1 -> bus_creator/2  "HybVehMde_D_ActlMntr"
  Inv1Ain_I_ActlMntr/1 -> bus_creator/3  "Inv1Ain_I_ActlMntr"
  Mtr2State_D_ActlMntr/1 -> bus_creator/4  "Mtr2State_D_ActlMntr"
  VehElRnge_L_Dsply/1 -> bus_creator/5  "VehElRnge_L_Dsply"

== system test_mdl/FD1_CAN_P702_GASD_MY21_DCV_V06/SOBDMC_HPCM_FD1/OTAPhysSOBDMCtoGWM_FD1 ==
  OTAPhysHPCMtoGWM_ECG : Constant
  bus_creator : BusCreator  Inputs=1
  port : Outport
  wires:
  bus_creator/1 -> port/1  "OTAPhysSOBDMCtoGWM_FD1"
  OTAPhysHPCMtoGWM_ECG/1 -> bus_creator/1  "OTAPhysHPCMtoGWM_ECG"

== system test_mdl/FD1_CAN_P702_GASD_MY21_DCV_V06/SOBDMC_HPCM_FD1/PARSEDHPCMtoGWM_ECG_FD1 ==
  PARSEDPhysHPCMtoGWM_ECG : Constant
  bus_creator : BusCreator  Inputs=1
  port : Outport
  wires:
  bus_creator/1 -> port/1  "PARSEDHPCMtoGWM_ECG_FD1"
  PARSEDPhysHPCMtoGWM_ECG/1 -> bus_creator/1  "PARSEDPhysHPCMtoGWM_ECG"

== system test_mdl/FD1_CAN_P702_GASD_MY21_DCV_V06/SOBDMC_HPCM_FD1/PARSEDPushSOBDMCtoGWM_FD1 ==
  PARSEDPhysHPCM2toGWM_ECG : Constant
  bus_creator : BusCreator  Inputs=1
  port : Outport
  wires:
  bus_creator/1 -> port/1  "PARSEDPushSOBDMCtoGWM_FD1"
  PARSEDPhysHPCM2toGWM_ECG/1 -> bus_creator/1  "PARSEDPhysHPCM2toGWM_ECG"

== system test_mdl/FD1_CAN_P702_GASD_MY21_DCV_V06/SOBDMC_HPCM_FD1/PreCond_Hev_Data1_FD1 ==
  BattChrgInhbt_D_Rq : Constant
  ChrgStat_D2_Dsply : Constant
  ChrgTMatch_B_Stat : Constant
  HvacPrecondAC_D_Rq : Constant
  HvacPrecondBlwr2_D_Rq : Constant
  HvacPrecondMode2_D_Rq : Constant
  HvacPrecondRecirc_D_Rq : Constant
  HvacPrecond_Te_Rq : Constant
  bus_creator : BusCreator  Inputs=8
  port : Outport
  wires:
  bus_creator/1 -> port/1  "PreCond_Hev_Data1_FD1"
  BattChrgInhbt_D_Rq/1 -> bus_creator/1  "BattChrgInhbt_D_Rq"
  ChrgStat_D2_Dsply/1 -> bus_creator/2  "ChrgStat_D2_Dsply"
  ChrgTMatch_B_Stat/1 -> bus_creator/3  "ChrgTMatch_B_Stat"
  HvacPrecondAC_D_Rq/1 -> bus_creator/4  "HvacPrecondAC_D_Rq"
  HvacPrecondBlwr2_D_Rq/1 -> bus_creator/5  "HvacPrecondBlwr2_D_Rq"
  HvacPrecondMode2_D_Rq/1 -> bus_creator/6  "HvacPrecondMode2_D_Rq"
  HvacPrecondRecirc_D_Rq/1 -> bus_creator/7  "HvacPrecondRecirc_D_Rq"
  HvacPrecond_Te_Rq/1 -> bus_creator/8  "HvacPrecond_Te_Rq"
